simulink model "TX_TUNE_DIGITALv4"  (R2024a)
settings: Solver=VariableStepAuto  StartTime=0.0  StopTime=0.5e-3  FixedStep=1e-9  RelTol=1e-3
values from neighbouring files (symbols this model uses):
  cnt_n_bits = 9    [TX_PM_MODEL_Setup.m]
  fH = 2*pi * (fin) / (2*pi - pi/2/N_PHASE_CYCLES)    (= 1066666.66667)    [TX_PM_MODEL_Setup.m]
  fin = 1e6    (= 1000000)    [TX_PM_MODEL_Setup.m]
  fL = 2*pi * (fin) / (2*pi + pi/2/N_PHASE_CYCLES)    (= 941176.470588)    [TX_PM_MODEL_Setup.m]
  VDD = 5    [Oscillator_Setup.m]    (also in TX_PM_MODEL_Setup.m = 10)
libraries: MyLib x3, simulink x1, dspsigops x1
settings Model: Creator=cian.odonnell  LastModifiedBy=ciano
settings SolverCC: EnableFixedStepZeroCrossing=on

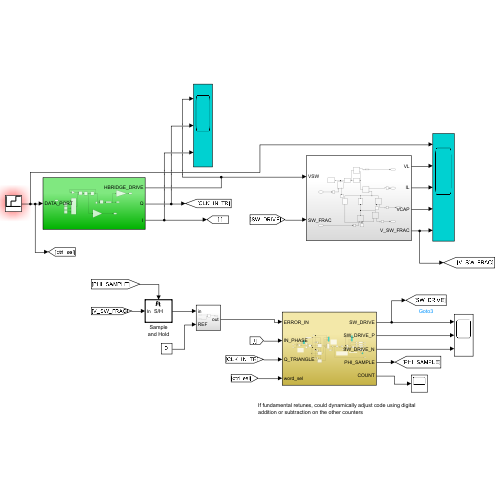
[thumbnail: Simulink's stored preview of the top-level diagram]
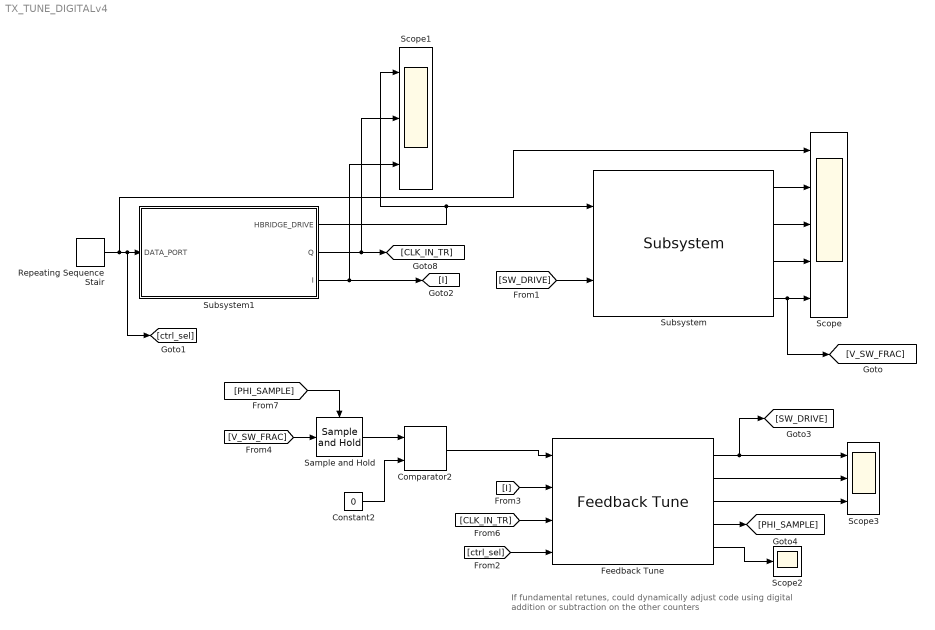
== system TX_TUNE_DIGITALv4 ==
  note: If fundamental retunes, could dynamically adjust code using digital
      | addition or subtraction on the other counters
  Comparator2 : MyLib/Comparator2  SystemSampleTime=-1  VariantActivationTime=update diagram  AllowFlexibleInterface=on  Latency=0  AutoFrameSizeCalculation=off
  Constant2 : Constant  Value=0
  Feedback Tune : MyLib/Feedback Tune  SystemSampleTime=-1  VariantActivationTime=update diagram  AllowFlexibleInterface=on  Latency=0  AutoFrameSizeCalculation=off
  Repeating Sequence Stair : simulink/Sources/Repeating Sequence Stair  OutValues=[0 1 2].'  tsamp=20/fin  OutMin=[]  OutMax=[]  OutDataTypeStr=double  OutputDataTypeScalingMode=double  OutDataType=fixdt(0,8)  ConRadixGroup=Best Precision: Vector-wise  OutScaling=2^-12
  Sample and Hold : dspsigops/Sample and Hold  trig=Either edge  initCond=0  latchinput=off
  Scope : Scope  NumInputPorts=5
  Scope1 : Scope  NumInputPorts=3
  Scope2 : Scope
  Scope3 : Scope  NumInputPorts=3
  Subsystem : MyLib/Subsystem  SystemSampleTime=-1  VariantActivationTime=update diagram  AllowFlexibleInterface=on  Latency=0  AutoFrameSizeCalculation=off
  Subsystem1 : Subsystem
  wires:
  Subsystem/1 -> Scope/2
  Subsystem/2 -> Scope/3
  Subsystem/3 -> Scope/4
  Subsystem/4 -> [V_SW_FRAC], Scope/5
  Feedback Tune/3 -> Scope3/3
  [I] -> Feedback Tune/2
  [CLK_IN_TR] -> Feedback Tune/3
  Comparator2/1 -> Feedback Tune/1
  Feedback Tune/1 -> Scope3/1, [SW_DRIVE]
  [SW_DRIVE] -> Subsystem/2
  [ctrl_sel] -> Feedback Tune/4
  [V_SW_FRAC] -> Sample and Hold/1
  Sample and Hold/1 -> Comparator2/1
  Constant2/1 -> Comparator2/2
  Feedback Tune/4 -> [PHI_SAMPLE]
  [PHI_SAMPLE] -> Sample and Hold/Trigger
  Subsystem1/2(Q) -> Scope1/2, [CLK_IN_TR]
  Subsystem1/3(I) -> Scope1/3, [I]
  Subsystem1/1(HBRIDGE_DRIVE) -> Subsystem/1, Scope1/1
  Repeating Sequence Stair/1 -> Scope/1, [ctrl_sel], Subsystem1/1(DATA_PORT)
  Feedback Tune/5 -> Scope2/1
  Feedback Tune/2 -> Scope3/2

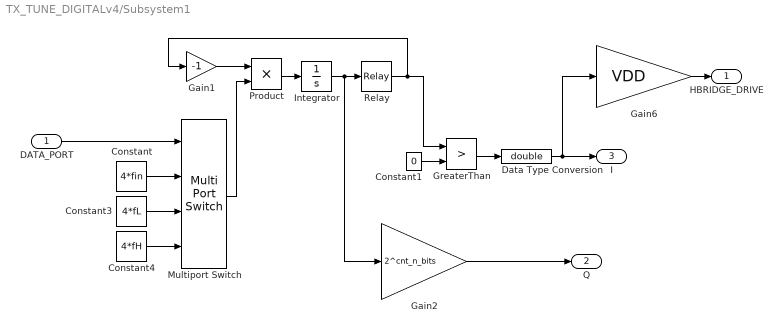
== system TX_TUNE_DIGITALv4/Subsystem1 ==
  DATA_PORT : Inport
  Constant : Constant  Value=4*fin
  Constant1 : Constant  Value=0
  Constant3 : Constant  Value=4*fL
  Constant4 : Constant  Value=4*fH
  Data Type Conversion : DataTypeConversion  OutDataTypeStr=double  SaturateOnIntegerOverflow=off  RndMeth=Floor
  Gain1 : Gain  Gain=-1
  Gain2 : Gain  Gain=2^cnt_n_bits
  Gain6 : Gain  Gain=VDD
  GreaterThan : RelationalOperator  Operator=>  OutDataTypeStr=boolean  RndMeth=Simplest  InputSameDT=off
  Integrator : Integrator
  Multiport Switch : MultiPortSwitch  DataPortOrder=Zero-based contiguous  zeroidx=on  SaturateOnIntegerOverflow=off  InputSameDT=off
  Product : Product
  Relay : Relay  OnSwitchValue=1  OffSwitchValue=-1  OffOutputValue=-1
  HBRIDGE_DRIVE : Outport
  Q : Outport  Port=2
  I : Outport  Port=3
  wires:
  Gain1/1 -> Product/1
  Multiport Switch/1 -> Product/2
  Constant/1 -> Multiport Switch/2
  Constant4/1 -> Multiport Switch/4
  Integrator/1 -> Gain2/1, Relay/1
  Constant3/1 -> Multiport Switch/3
  Product/1 -> Integrator/1
  Gain2/1 -> Q/1
  DATA_PORT/1 -> Multiport Switch/1
  Relay/1 -> GreaterThan/1, Gain1/1
  Data Type Conversion/1 -> Gain6/1, I/1
  GreaterThan/1 -> Data Type Conversion/1
  Constant1/1 -> GreaterThan/2
  Gain6/1 -> HBRIDGE_DRIVE/1
